simulink model "PTSD"  (R2020a)
settings: Solver=VariableStepAuto  StartTime=0.0  StopTime=10  RelTol=1e-3
undefined symbols (not defined in the file): fs, refractory
libraries: simulink x6, dspstat3 x2, dspswit3 x1, dspfdesign x1, hdlsllib x1
settings Model: Creator=sbuccelli  LastModifiedBy=diflo

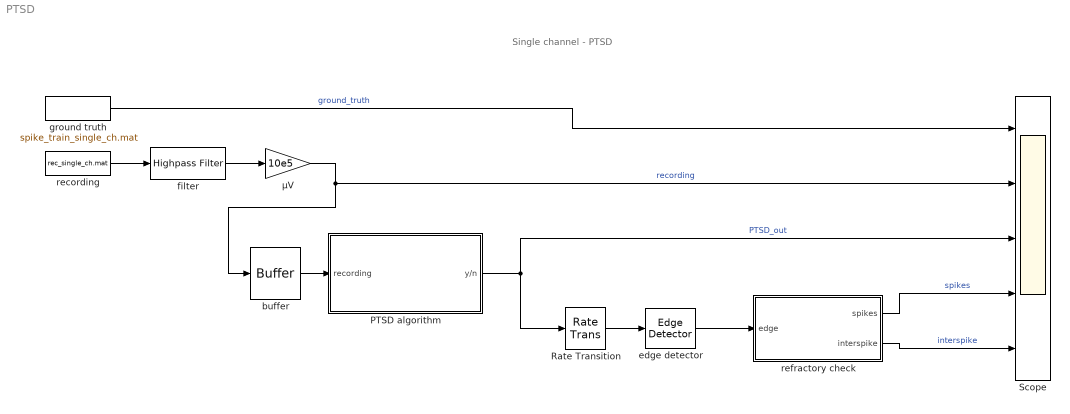
== system PTSD ==
  note: Single channel - PTSD
  PTSD algorithm : Subsystem
  Rate Transition : RateTransition  OutPortSampleTime=1/32000
  Scope : Scope  NumInputPorts=5
  buffer : Buffer  N=33  V=32  OutputFrames=off
  edge detector : dspswit3/Edge Detector  InputProcessing=Columns as channels (frame based)
      settings: SourceProductBaseCode=DS
  filter : dspfdesign/Highpass Filter  FilterType=IIR  DesignForMinimumOrder=off  FilterOrder=3  StopbandFrequency=1  PassbandFrequency=300  StopbandAttenuation=80  PassbandRipple=0.1  InheritSampleRate=off  SampleRate=30000  SimulateUsing=Interpreted execution  roundingMode=Floor  coeffsDataTypeStr=fixdt(1,16)
  ground truth : FromFile  FileName=spike_train_single_ch.mat  SampleTime=1/fs
  recording : FromFile  FileName=rec_single_ch.mat  SampleTime=1/fs
  refractory check : Subsystem
  μV : Gain  Gain=10e5
  wires:
  recording/1 -> filter/1
  Rate Transition/1 -> edge detector/1
  filter/1 -> μV/1
  μV/1 -> Scope/2, buffer/1  "recording"
  buffer/1 -> PTSD algorithm/1(recording)
  PTSD algorithm/1(y/n) -> Rate Transition/1, Scope/3  "PTSD_out"
  edge detector/1 -> refractory check/1(" edge  ")
  refractory check/1(" spikes") -> Scope/4  "spikes"
  refractory check/2(interspike) -> Scope/5  "interspike"
  ground truth/1 -> Scope/1  "ground_truth"

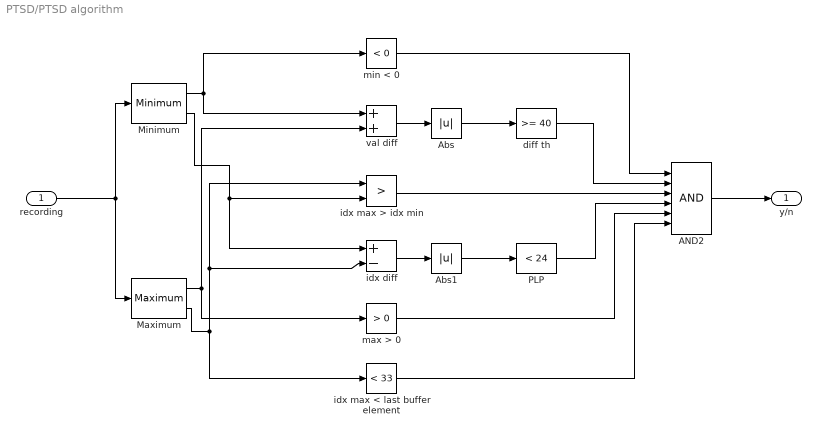
== system PTSD/PTSD algorithm ==
  recording : Inport
  AND2 : Logic  Inputs=6  IconShape=distinctive  AllPortsSameDT=off  OutDataTypeStr=boolean
  Abs : Abs
  Abs1 : Abs
  Maximum : dspstat3/Maximum  operation=maximum  fcn=Value and Index  indexBase=One  operateOver=Each column  Dimension=1  InputProcessing=Columns as channels (frame based)  reset=None  roiEnable=off  roiType=Rectangles  roiPortion=Entire ROI  roiOutput=Individual statistics for each ROI  roiFlag=off  roundingMode=Floor  overflowMode=off  accumDataTypeStr=Inherit: Same as product output  accumLastDataTypeStr=Inherit: Same as product output
  Minimum : dspstat3/Minimum  operation=minimum  fcn=Value and Index  indexBase=One  operateOver=Each column  Dimension=1  InputProcessing=Columns as channels (frame based)  reset=None  roiEnable=off  roiType=Rectangles  roiPortion=Entire ROI  roiOutput=Individual statistics for each ROI  roiFlag=off  roundingMode=Floor  overflowMode=off
      settings: SourceProductBaseCode=DS
  PLP : simulink/Logic and Bit Operations/Compare To Constant  relop=<  const=24  OutDataTypeStr=boolean
  diff th : simulink/Logic and Bit Operations/Compare To Constant  relop=>=  const=40  OutDataTypeStr=boolean
  idx diff : Sum  Inputs=+-
  idx max < last buffer element : simulink/Logic and Bit Operations/Compare To Constant  relop=<  const=33  OutDataTypeStr=boolean
  idx max > idx min : RelationalOperator  Operator=>  OutDataTypeStr=boolean  RndMeth=Simplest
  max > 0 : simulink/Logic and Bit Operations/Compare To Constant  relop=>  const=0  OutDataTypeStr=boolean
  min < 0 : simulink/Logic and Bit Operations/Compare To Constant  relop=<  const=0  OutDataTypeStr=boolean
  val diff : Sum
  y/n : Outport
  wires:
  Minimum/2 -> idx diff/1, idx max > idx min/2
  Maximum/2 -> idx max > idx min/1, idx diff/2, idx max < last buffer element/1
  val diff/1 -> Abs/1
  Maximum/1 -> val diff/2, max > 0/1
  Abs1/1 -> PLP/1
  recording/1 -> Maximum/1, Minimum/1
  Abs/1 -> diff th/1
  idx diff/1 -> Abs1/1
  Minimum/1 -> val diff/1, min < 0/1
  min < 0/1 -> AND2/1
  diff th/1 -> AND2/2
  idx max > idx min/1 -> AND2/3
  PLP/1 -> AND2/4
  max > 0/1 -> AND2/5
  idx max < last buffer element/1 -> AND2/6
  AND2/1 -> y/n/1

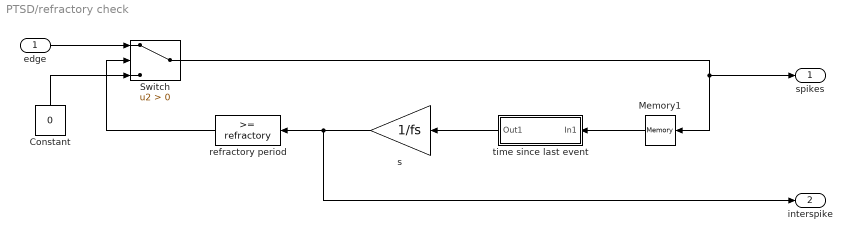
== system PTSD/refractory check ==
  " edge  " : Inport
  Constant : Constant  Value=0
  Memory1 : Memory  InheritSampleTime=on
  Switch : Switch  Criteria=u2 > Threshold
  refractory period : simulink/Logic and Bit Operations/Compare To Constant  relop=>=  const=refractory  OutDataTypeStr=boolean
  s : Gain  Gain=1/fs  ParamDataTypeStr=double
  time since last event : Subsystem
  " spikes" : Outport
  interspike : Outport  Port=2
  wires:
  " edge  "/1 -> Switch/1
  Memory1/1 -> time since last event/1(In1)
  time since last event/1(Out1) -> s/1
  Constant/1 -> Switch/3
  s/1 -> refractory period/1, interspike/1
  Switch/1 -> " spikes"/1, Memory1/1
  refractory period/1 -> Switch/2

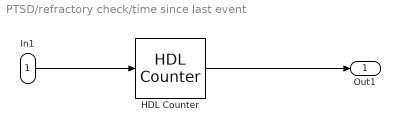
== system PTSD/refractory check/time since last event ==
  In1 : Inport
  HDL Counter : hdlsllib/Sources/HDL Counter  CountType=Free running  CountInit=1  CountStep=1  CountMax=25  CountFromType=Initial value  CountFrom=1  CountResetPort=on  CountLoadPort=off  CountEnbPort=off  CountDirPort=off  CountDataType=Unsigned  CountWordLen=32  CountFracLen=0  CountSampTime=1
  Out1 : Outport
  wires:
  In1/1 -> HDL Counter/1
  HDL Counter/1 -> Out1/1
